simulink model "Calculator_graphical_function"  (R2018a)
settings: Solver=FixedStepDiscrete  StartTime=0.0  StopTime=10.0  RelTol=1e-3
settings Model: Creator=Moataz  LastModifiedBy=Moataz
settings OptimizationCC: DefaultParameterBehavior=Inlined  EnhancedBackFolding=on  PassReuseOutputArgsAs=Individual arguments  OptimizeBlockOrder=speed  DifferentSizesBufferReuse=on  OptimizationCustomize=off
settings DebuggingCC: ParameterTunabilityLossMsg=error
settings SFSimCC: MATLABDynamicMemAlloc=off
settings RTWCC: SystemTargetFile=ert.tlc  GenCodeOnly=on  TemplateMakefile=ert_default_tmf  GenerateReport=on  IncludeHyperlinkInReport=on  LaunchReport=on  GenerateTraceInfo=on  GenerateTraceReport=on  GenerateTraceReportSl=on  GenerateTraceReportSf=on  GenerateTraceReportEml=on
settings CodeAppCC: ForceParamTrailComments=on  IgnoreCustomStorageClasses=off  OperatorAnnotations=on  SimulinkDataObjDesc=on  SFDataObjDesc=on  InsertBlockDesc=on
settings ERTTargetCC: TargetLangStandard=C99 (ISO)  GenerateSampleERTMain=on  InlinedParameterPlacement=NonHierarchical  ERTCustomFileTemplate=example_file_process.tlc

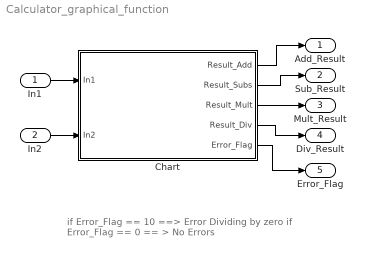
== system Calculator_graphical_function ==
  note: if Error_Flag == 10 ==> Error Dividing by zero
      | if Error_Flag == 0 == > No Errors
  In1 : Inport
  In2 : Inport  Port=2
  Chart : Stateflow chart  TreatAsAtomicUnit=on
  Add_Result : Outport
  Sub_Result : Outport  Port=2
  Mult_Result : Outport  Port=3
  Div_Result : Outport  Port=4
  Error_Flag : Outport  Port=5
  wires:
  In1/1 -> Chart/1(In1)
  In2/1 -> Chart/2(In2)
  Chart/1(Result_Add) -> Add_Result/1
  Chart/3(Result_Mult) -> Mult_Result/1
  Chart/2(Result_Subs) -> Sub_Result/1
  Chart/4(Result_Div) -> Div_Result/1
  Chart/5(Error_Flag) -> Error_Flag/1

== stateflow chart Calculator_graphical_function/Chart ==
  state Add(In1,In2) [function]
    (default) -> (junction 11) : {Result_Add = In1+In2;}
  state Sub(In1,In2) [function]
    (default) -> (junction 20) : {Result_Subs = In1-In2;}
  state Mult(In1,In2) [function]
    (default) -> (junction 25) : {Result_Mult = In1*In2;}
  state Div(In1,In2) [function]
    (default) -> (junction 46) : /* Division */
    (junction 46) -> (junction 47) [order 1] : [In2!=0]
    (junction 46) -> (junction 48) [order 2] : {Error_Flag=10;}
    (junction 47) -> (junction 49) : {Result_Div = In1/In2;}
    (junction 49) -> (junction 48)
    (junction 48) -> (junction 50)
  (default) -> (junction 4) : {Add(In1,In2);
      | Sub(In1,In2);
      | Mult(In1,In2);
      | Div(In1,In2);
      | }
  data: In1 function_input double; In2 function_input double; In1 function_input double; In2 function_input double; In1 function_input double; In2 function_input double; In1 function_input double; In2 function_input double; In1 input int16; In2 input int16; Result_Add output int16; Result_Subs output int16; Result_Mult output int16; Result_Div output double; Error_Flag output int16
